simulink library "lib_Convection_ChurchillBernstein"  (R2015a)
settings: Solver=ode45  StartTime=0.0  StopTime=10.0  RelTol=1e-3
libraries: simulink x1
settings Model: Creator=jlkratz  LastModifiedBy=jlkratz

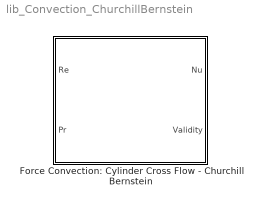
== system lib_Convection_ChurchillBernstein ==
  Force Convection: Cylinder Cross Flow - Churchill Bernstein : Subsystem  mask(TSAT: Cylinder Cross Flow - Churchill & Bernstein){}
      mask help:
      | This block estimates the average Nusselt number of an external flow over an isothermal cylinder. The correlation employed was developed by Churchill and Bernstein. It is a single comprehensive equtaion that covers a wide range of Reynolds number (Re) and Prandtl number (Pr). The Reynolds number should be calculated based on the cylinder diameter. All properties of the fluid should be evaluated at the film temperature. The correlation is subject to the following restrictions:
      |
      | Re*Pr >= 0.2
      |
      | For more information see the block help menu.
      mask Help: web(which('Convection_TSAT_CylinderCrossFlowChurchillBern.html'),'-helpbrowser')

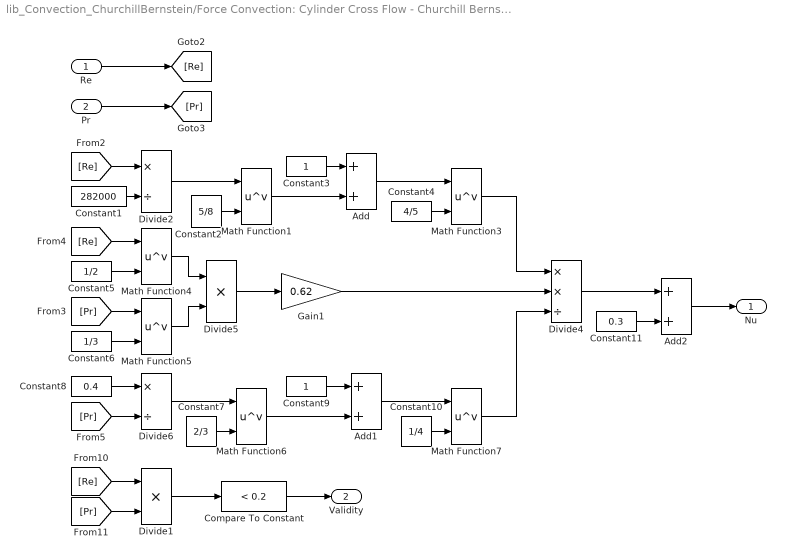
== system lib_Convection_ChurchillBernstein/Force Convection: Cylinder Cross Flow - Churchill Bernstein ==
  Re : Inport
  Pr : Inport  Port=2
  Add : Sum
  Add1 : Sum
  Add2 : Sum
  Compare To Constant : simulink/Logic and Bit Operations/Compare To Constant  relop=<  const=0.2  OutDataTypeStr=boolean
  Constant1 : Constant  Value=282000
  Constant10 : Constant  Value=1/4
  Constant11 : Constant  Value=0.3
  Constant2 : Constant  Value=5/8
  Constant3 : Constant
  Constant4 : Constant  Value=4/5
  Constant5 : Constant  Value=1/2
  Constant6 : Constant  Value=1/3
  Constant7 : Constant  Value=2/3
  Constant8 : Constant  Value=0.4
  Constant9 : Constant
  Divide1 : Product  Inputs=**
  Divide2 : Product  Inputs=*/
  Divide4 : Product  Inputs=**/
  Divide5 : Product  Inputs=**
  Divide6 : Product  Inputs=*/
  Gain1 : Gain  Gain=0.62
  Math Function{1,3..7} (6 alike) : Math  Operator=pow  SaturateOnIntegerOverflow=on
  Nu : Outport
  Validity : Outport  Port=2
  wires:
  Compare To Constant/1 -> Validity/1
  Divide1/1 -> Compare To Constant/1
  [Pr] -> Divide1/2
  [Re] -> Divide1/1
  Add2/1 -> Nu/1
  Constant11/1 -> Add2/2
  Divide4/1 -> Add2/1
  Math Function7/1 -> Divide4/3
  Gain1/1 -> Divide4/2
  Math Function3/1 -> Divide4/1
  Constant10/1 -> Math Function7/2
  Add1/1 -> Math Function7/1
  Math Function6/1 -> Add1/2
  Constant9/1 -> Add1/1
  Constant8/1 -> Divide6/1
  [Pr] -> Divide6/2
  Constant7/1 -> Math Function6/2
  Divide6/1 -> Math Function6/1
  [Pr] -> Math Function5/1
  [Re] -> Math Function4/1
  Divide5/1 -> Gain1/1
  Math Function5/1 -> Divide5/2
  Math Function4/1 -> Divide5/1
  Constant6/1 -> Math Function5/2
  Constant5/1 -> Math Function4/2
  Constant4/1 -> Math Function3/2
  Add/1 -> Math Function3/1
  Constant3/1 -> Add/1
  Math Function1/1 -> Add/2
  Divide2/1 -> Math Function1/1
  Constant1/1 -> Divide2/2
  [Re] -> Divide2/1
  Pr/1 -> [Pr]
  Re/1 -> [Re]
  Constant2/1 -> Math Function1/2
